simulink model "SquareWaveSumOfSineWaves_MathFunction_2"  (R2015b)
settings: Solver=VariableStepAuto  StartTime=0.0  StopTime=10.0  MaxStep=0.001  MinStep=0.001  RelTol=1e-3
settings Model: Creator=mihai.ciobanu  LastModifiedBy=mihai.ciobanu

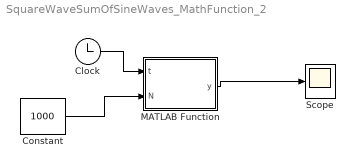
== system SquareWaveSumOfSineWaves_MathFunction_2 ==
  Clock : Clock
  Constant : Constant  Value=1000
  MATLAB Function : MATLAB Function  TreatAsAtomicUnit=on
  Scope : Scope
  wires:
  Constant/1 -> MATLAB Function/2(N)
  Clock/1 -> MATLAB Function/1(t)
  MATLAB Function/1(y) -> Scope/1

== matlab function SquareWaveSumOfSineWaves_MathFunction_2/MATLAB Function ==
  data: t input; N input; y output
function y = fcn(t, N)
%#codegen
y=0;
for K=1:2:N
    %Frad = K/(2*pi);
    %sum = sum+ K*sin(Frad*t);    
    y = y+ (1/K)*sin(K*t);    
end
